simulink model "provaAttitude"  (R2023b)
settings: Solver=ode4  StartTime=t0  StopTime=tf  FixedStep=t_step  RelTol=1e-3
values from neighbouring files (symbols this model uses):
  A = 1e-2.*[6, 6, 6, 6, 4, 4, 12, 12, 12, 12]'    [provaAttitudeCode.m]
  A1 = ones(length(BODY),1)    [provaAttitudeCode.m]
  alpha = alpha/norm(alpha)    [provaAttitudeCode.m]
  BODY = [1, 0, 0 ... (first row only)    [provaAttitudeCode.m]
  c = 3e8    (= 300000000)    [provaAttitudeCode.m]
  DCM_eci_per = rotationMatrix(rad2deg(i),rad2deg(OM), rad2deg(om))    [provaAttitudeCode.m]
  e = 0.0001    [provaAttitudeCode.m]
  epsilon = deg2rad(23.45)    [provaAttitudeCode.m]
  Fe = 1358    [provaAttitudeCode.m]
  FS = 800e-9    (= 8e-07)    [provaAttitudeCode.m]
  H0 = 1e-9.*[-29404.8 -1450.9 4652.5]'    [provaAttitudeCode.m]
  horizon_cone_limit = deg2rad(67)    [provaAttitudeCode.m]
  i = deg2rad(90)    [provaAttitudeCode.m]
  I = [Ix, 0, 0; 0, Iy, 0; 0, 0, Iz]    [provaAttitudeCode.m]
  I_inv = inv(I)    [provaAttitudeCode.m]
  inc_tot = sqrt(inc_lin^2 + inc_acc^2)    [provaAttitudeCode.m]
  j_b = [0.01 0.05 0.01]'    [provaAttitudeCode.m]
  MJD2000_initial = date2mjd2000(date0)    [provaAttitudeCode.m]
  mu_E = astroConstants(13)    [provaAttitudeCode.m]
  n_e = sqrt(mu_E/a^3)    [provaAttitudeCode.m]
  p = a*(1-e^2)    [provaAttitudeCode.m]
  pd = 0.1.*A1    [provaAttitudeCode.m]
  ps = [0.5, 0.5, 0.5, 0.5, 0.5, 0.5, 0.1, 0.1, 0.1, 0.1]'    [provaAttitudeCode.m]
  q0 = [0 0 0 1]    [provaAttitudeCode.m]
  r1 = r(:,1) + CMC_position(1).*ones(10,1)    [provaAttitudeCode.m]
  r2 = r(:,2) + CMC_position(2).*ones(10,1)    [provaAttitudeCode.m]
  r3 = r(:,3)+ CMC_position(3).*ones(10,1)    [provaAttitudeCode.m]
  R_E = astroConstants(23)    [provaAttitudeCode.m]
  th0 = deg2rad(0)    [provaAttitudeCode.m]
  ts_sensor = t_step    (= 0.01)    [provaAttitudeCode.m]
  w0 = [wx0 wy0 wz0]'    [provaAttitudeCode.m]
  w_E = deg2rad(15.04)/60/60    [provaAttitudeCode.m]
  w_r = 0    [provaAttitudeCode.m]
libraries: matrix_library x16, dspindex x6, simulink_extras x4, simulink x3, aerolibutil x2
(part 1 of 2)
settings Model: Creator=samue  LastModifiedBy=samue

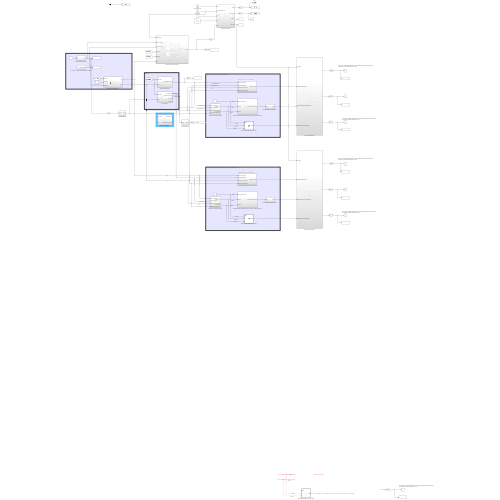
[thumbnail: Simulink's stored preview of the top-level diagram]
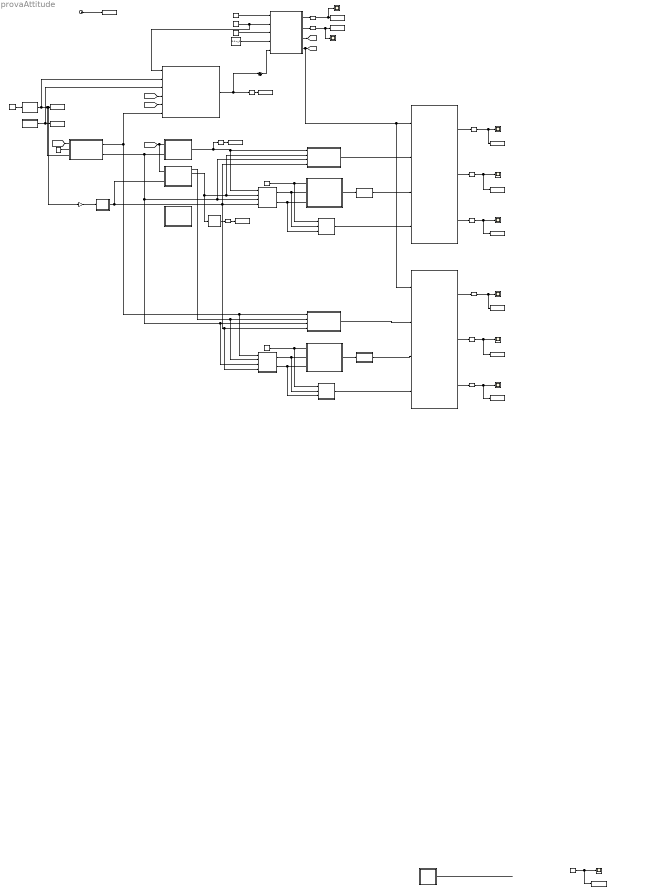
== system provaAttitude ==
  note: COMPARISON ATTITUDE DETERMINATION
  note: SENSOR
  note: Error from the real DCM and DCM att Det. If we eliminate the disturbance, sample holder and saturation we obtain estimate error of 1e-15
  note: Enviroment
  note: Error from the real DCM and DCM att Det. If we eliminate the disturbance, sample holder and saturation we obtain estimate error of 1e-11
  note: inside the block there is a normalisation
  note: UnPERTURBED CASE COMPARISON ATTITUDE DETERMINATION
  note: Error from the real DCM and DCM att Det. If we eliminate the disturbance, sample holder and saturation we obtain estimate error of 1e-11
  note: Error from the real DCM and DCM att Det. If we eliminate the disturbance, sample holder and saturation we obtain estimate error of 1e-15
  note: inside the block there is a normalisation
  note: Error from the real DCM and DCM att Det. If we eliminate the disturbance, sample holder and saturation we obtain estimate error of 1e-11
  Attitude determination algebric Method with 2 sensor : Subsystem
  Attitude determination algebric Method with 2 sensor1 : Subsystem
  Calculation of disturbance torque : Subsystem
  Clock : Clock
  Comparison (sottrazione) : Subsystem
  Comparison (sottrazione)1 : Subsystem
  Constant : Constant  Value=I_inv
  Constant1 : Constant  Value=alpha
  Constant2 : Constant  Value=[0,0,w_r]
  Constant3 : Constant  Value=alpha
  Constant4 : Constant  Value=th0
  Create matrix to statistical method : Subsystem
  Create matrix to statistical method1 : Subsystem
  DCM composition from quaternions 1 : Subsystem  AncestorBlock=LibrarySAD5/DCM composition from quaternions
  DCM composition from quaternions 2 : Subsystem  AncestorBlock=LibrarySAD5/DCM composition from quaternions
  Dipol Model of Magnetic Field : Subsystem
  Dynamics e Kinematics : Subsystem
  Gain : Gain  Gain=-1
  Horizon Sensor : Subsystem
  Inertia Matrix : Constant  Value=I  VectorParams1D=off
  Initial Condition W : Constant  Value=w0
  MAG-3  Magnetometer : Subsystem
  Normalize Vector1 : Subsystem
  Normalize Vector3 : Subsystem
  Ouput DCM with gibbs vector (ver slide) : MATLAB Function  TreatAsAtomicUnit=on
  Ouput DCM with gibbs vector (ver slide)1 : MATLAB Function  TreatAsAtomicUnit=on
  Ouput DCM with gibbs vector (ver slide)3 : MATLAB Function  TreatAsAtomicUnit=on
  Reshape{,1..10,17} (12 alike) : Reshape
  Scope{,1..7,10} (9 alike) : Scope
  "Statistical methods attitude determination (quaternion  Wabha’s problem) " : Subsystem
  Statistical methods attitude determination (quaternion  Wabha’s problem) 1 : Subsystem
  Sum : Sum  Inputs=|++
  Sun Position in Earth Centred Equatorial Inertial RF : Subsystem
  Sun sensor (Da fare) : Subsystem
  To Workspace : ToWorkspace  VariableName=r_n  SampleTime=-1
  To Workspace1 : ToWorkspace  VariableName=s_n  SampleTime=-1
  To Workspace10 : ToWorkspace  VariableName=erro_statistic_quat_unp  SampleTime=-1
  To Workspace11 : ToWorkspace  VariableName=erro_statistic_gibb_unp  SampleTime=-1
  To Workspace12 : ToWorkspace  VariableName=b_sensor  SampleTime=-1
  To Workspace13 : ToWorkspace  VariableName=sun_sensor  SampleTime=-1
  To Workspace15 : ToWorkspace  VariableName=erro_statistic_gibb_unp1  SampleTime=-1
  To Workspace2 : ToWorkspace  VariableName=wb  SampleTime=-1
  To Workspace3 : ToWorkspace  VariableName=M_dist  SaveFormat=Timeseries  SampleTime=-1
  To Workspace4 : ToWorkspace  VariableName=w  SampleTime=-1
  To Workspace5 : ToWorkspace  VariableName=erro_algebric_met  SampleTime=-1
  To Workspace6 : ToWorkspace  VariableName=erro_statistic_quat  SampleTime=-1
  To Workspace7 : ToWorkspace  VariableName=t  SampleTime=-1
  To Workspace8 : ToWorkspace  VariableName=erro_statistic_gibb  SampleTime=-1
  To Workspace9 : ToWorkspace  VariableName=erro_algebric_met_unp  SampleTime=-1
  "[g0_1, g1_1, h1_1]" : Constant  Value=H0
  two-body Keplerian dynamics : Subsystem
  wires:
  Constant2/1 -> Dynamics e Kinematics/4(w_r)
  Constant1/1 -> "Statistical methods attitude determination (quaternion  Wabha’s problem) "/1(alpha (weigh of sensor)), Ouput DCM with gibbs vector (ver slide)/1(alpha)  "alpha"
  two-body Keplerian dynamics/1(r_n) -> Calculation of disturbance torque/2(EarthSat_n vector), To Workspace/1, Gain/1, Dipol Model of Magnetic Field/3(EarthSat_n)
  [DCM_BN] -> Dipol Model of Magnetic Field/1(DCM_B/N)
  Sun Position in Earth Centred Equatorial Inertial RF/1(S_EarthSun_N) -> To Workspace1/1, Calculation of disturbance torque/3(SunEarth_n vector)  "S_n"
  Dipol Model of Magnetic Field/2(b_N) -> MAG-3  Magnetometer/2(B_N), Create matrix to statistical method/3(Reference1 (Inertial frame)), Attitude determination algebric Method with 2 sensor/3(Reference1 (Inertial frame)), Create matrix to statistical method1/3(Reference1 (Inertial frame)), Attitude determination algebric Method with 2 sensor1/3(Reference1 (Inertial frame))  "B_n"
  Reshape1/1 -> Scope7/1, To Workspace4/1
  Dipol Model of Magnetic Field/1(b_b) -> Create matrix to statistical method1/1(Sensor1 (body frame)), Attitude determination algebric Method with 2 sensor1/1(Sensor1 (body frame)), Calculation of disturbance torque/6(B_b)  "B_b"
  "[g0_1, g1_1, h1_1]"/1 -> Dipol Model of Magnetic Field/2(H0 vector)
  "Statistical methods attitude determination (quaternion  Wabha’s problem) "/1(q in quaternion (scalar last)) -> DCM composition from quaternions 1/1(q(4x1))
  [DCM_BN] -> Calculation of disturbance torque/5(DCM_B/N)
  [DCM_BL] -> Calculation of disturbance torque/4(DCM_B/L)
  MAG-3  Magnetometer/1(B_b perturbed sensor) -> Reshape9/1, Create matrix to statistical method/1(Sensor1 (body frame)), Attitude determination algebric Method with 2 sensor/1(Sensor1 (body frame))  "B_b perturbed sensor"
  [DCM_BN] -> Horizon Sensor/1(DCM_B/N), MAG-3  Magnetometer/1(DCM_B/N)
  Constant/1 -> Dynamics e Kinematics/3(I_inv)
  Calculation of disturbance torque/1(M_dist) -> Sum/1, Reshape2/1
  Constant4/1 -> two-body Keplerian dynamics/1(th0)
  Dynamics e Kinematics/1(Omega) -> Reshape1/1
  Clock/1 -> To Workspace7/1
  Reshape2/1 -> To Workspace3/1
  Initial Condition W/1 -> Dynamics e Kinematics/1(w0)
  Dynamics e Kinematics/3(DCM_B/L) -> [DCM_BL]
  Dynamics e Kinematics/2(Ang Vel Error) -> Reshape/1
  Inertia Matrix/1 -> Calculation of disturbance torque/1(Inertia Matrix), Dynamics e Kinematics/2("Principal Inertia Vector ")
  Reshape/1 -> Scope/1, To Workspace2/1
  Create matrix to statistical method/1(S matrix (body)) -> "Statistical methods attitude determination (quaternion  Wabha’s problem) "/2(s matrix), Ouput DCM with gibbs vector (ver slide)/2(s)  "S matrix"
  Create matrix to statistical method/2(V matrix (inertia)) -> "Statistical methods attitude determination (quaternion  Wabha’s problem) "/3(v matrix), Ouput DCM with gibbs vector (ver slide)/3(v)  "V matrix"
  Attitude determination algebric Method with 2 sensor/1(DCM_B/N  Att Det) -> Comparison (sottrazione)/2(DCM from Algebric method)
  DCM composition from quaternions 1/1(DCM) -> Comparison (sottrazione)/3("DCM from Statistic method (quaternion) ")
  Ouput DCM with gibbs vector (ver slide)/1(DCM) -> Comparison (sottrazione)/4("DCM from Statistic method (gibbs) ")
  Comparison (sottrazione)/1(Out1) -> Reshape3/1
  Comparison (sottrazione)/2(Out2) -> Reshape4/1
  Comparison (sottrazione)/3(Out3) -> Reshape5/1
  Reshape3/1 -> To Workspace5/1, Scope3/1
  Reshape4/1 -> To Workspace6/1, Scope2/1
  Reshape5/1 -> To Workspace8/1, Scope1/1
  Create matrix to statistical method1/1(S matrix (body)) -> Statistical methods attitude determination (quaternion  Wabha’s problem) 1/2(s matrix), Ouput DCM with gibbs vector (ver slide)1/2(s)  "S matrix"
  Create matrix to statistical method1/2(V matrix (inertia)) -> Statistical methods attitude determination (quaternion  Wabha’s problem) 1/3(v matrix), Ouput DCM with gibbs vector (ver slide)1/3(v)  "V matrix"
  Comparison (sottrazione)1/3(Out3) -> Reshape8/1
  Dynamics e Kinematics/4(DCM_B/N) -> Comparison (sottrazione)1/1(True DCM), Comparison (sottrazione)/1(True DCM), [DCM_BN]
  Attitude determination algebric Method with 2 sensor1/1(DCM_B/N  Att Det) -> Comparison (sottrazione)1/2(DCM from Algebric method)
  Comparison (sottrazione)1/2(Out2) -> Reshape7/1
  Ouput DCM with gibbs vector (ver slide)1/1(DCM) -> Comparison (sottrazione)1/4("DCM from Statistic method (gibbs) ")
  DCM composition from quaternions 2/1(DCM) -> Comparison (sottrazione)1/3("DCM from Statistic method (quaternion) ")
  Comparison (sottrazione)1/1(Out1) -> Reshape6/1
  Reshape7/1 -> To Workspace10/1, Scope5/1
  Constant3/1 -> Statistical methods attitude determination (quaternion  Wabha’s problem) 1/1(alpha (weigh of sensor)), Ouput DCM with gibbs vector (ver slide)1/1(alpha)  "alpha"
  Reshape6/1 -> To Workspace9/1, Scope6/1
  Statistical methods attitude determination (quaternion  Wabha’s problem) 1/1(q in quaternion (scalar last)) -> DCM composition from quaternions 2/1(q(4x1))
  Reshape8/1 -> To Workspace11/1, Scope4/1
  Reshape9/1 -> To Workspace12/1
  Horizon Sensor/2(Perturbed data Horizon) -> Normalize Vector1/1(Vector), Attitude determination algebric Method with 2 sensor/2(Sensor2 (body frame)), Create matrix to statistical method/2(Sensor2 (body frame))  "S_b perturbed sensor"
  Horizon Sensor/1(R_b unperturbed) -> Create matrix to statistical method1/2(Sensor2 (body frame)), Attitude determination algebric Method with 2 sensor1/2(Sensor2 (body frame))  "S_b unperturbed"
  Reshape10/1 -> To Workspace13/1
  Normalize Vector1/1(Versor) -> Reshape10/1
  Reshape17/1 -> To Workspace15/1, Scope10/1
  ? -> Ouput DCM with gibbs vector (ver slide)3/2(s)  "S matrix"
  ? -> ?
  ? -> Reshape17/1
  Ouput DCM with gibbs vector (ver slide)3/1(DCM) -> ?
  ? -> Ouput DCM with gibbs vector (ver slide)3/3(v)  "V matrix"
  Gain/1 -> Normalize Vector3/1(Vector)
  Normalize Vector3/1(Versor) -> Horizon Sensor/2(R_N), Create matrix to statistical method/4(Reference2 (Inertial frame)), Attitude determination algebric Method with 2 sensor/4(Reference2 (Inertial frame)), Create matrix to statistical method1/4(Reference2 (Inertial frame)), Attitude determination algebric Method with 2 sensor1/4(Reference2 (Inertial frame))
  Sum/1 -> Dynamics e Kinematics/5(M)

== system provaAttitude/Attitude determination algebric Method with 2 sensor ==
  note: 𝑉^(-1) = 𝑉';
      | 𝐴 = 𝑆𝑉^(-1) = 𝑆𝑉'
  note: 𝑣1 = 𝑎;
      | 𝑣2 = (𝑎 ∧ 𝑏)/|𝑎 ∧ 𝑏|;
      | 𝑣3 = 𝑎 ∧ 𝑣2
  note: S1 = 𝑝;
      | 𝑠2 = (𝑝 ∧ 𝑞)/(|𝑝 ∧ 𝑞|);
      | 𝑠3 = 𝑝 ∧ 𝑠2
  Sensor1 (body frame) : Inport
  Sensor2 (body frame) : Inport  Port=2
  Reference1 (Inertial frame) : Inport  Port=3
  Reference2 (Inertial frame) : Inport  Port=4
  Matrix Multiply : Product  Multiplication=Matrix(*)
  Normalize Vector1 : Subsystem
  Normalize Vector2 : Subsystem
  Normalize Vector3 : Subsystem
  Normalize Vector4 : Subsystem
  Subsystem : Subsystem
  Subsystem1 : Subsystem
  Transpose : Math  Operator=transpose
  DCM_B/N  Att Det : Outport
  wires:
  Sensor1 (body frame)/1 -> Normalize Vector2/1(Vector)  "q"
  Sensor2 (body frame)/1 -> Normalize Vector3/1(Vector)  "p"
  Subsystem/1("Matrix S Measurements ") -> Matrix Multiply/1  "Matrix S Measurements (body frame)"
  Normalize Vector2/1(Versor) -> Subsystem/1(versor p (body frame))
  Normalize Vector3/1(Versor) -> Subsystem/2(versor q (body frame))
  Normalize Vector1/1(Versor) -> Subsystem1/1(versor a (body frame))
  Reference2 (Inertial frame)/1 -> Normalize Vector4/1(Vector)  "b"
  Reference1 (Inertial frame)/1 -> Normalize Vector1/1(Vector)  "a"
  Subsystem1/1("Matrix V certain model ") -> Transpose/1  "Matrix V (inertial frame)"
  Normalize Vector4/1(Versor) -> Subsystem1/2(versor b (body frame))
  Matrix Multiply/1 -> DCM_B/N  Att Det/1  "DCM_B/N from attirude determination"
  Transpose/1 -> Matrix Multiply/2

== system provaAttitude/Attitude determination algebric Method with 2 sensor1 ==
  note: 𝑉^(-1) = 𝑉';
      | 𝐴 = 𝑆𝑉^(-1) = 𝑆𝑉'
  note: 𝑣1 = 𝑎;
      | 𝑣2 = (𝑎 ∧ 𝑏)/|𝑎 ∧ 𝑏|;
      | 𝑣3 = 𝑎 ∧ 𝑣2
  note: S1 = 𝑝;
      | 𝑠2 = (𝑝 ∧ 𝑞)/(|𝑝 ∧ 𝑞|);
      | 𝑠3 = 𝑝 ∧ 𝑠2
  Sensor1 (body frame) : Inport
  Sensor2 (body frame) : Inport  Port=2
  Reference1 (Inertial frame) : Inport  Port=3
  Reference2 (Inertial frame) : Inport  Port=4
  Matrix Multiply : Product  Multiplication=Matrix(*)
  Normalize Vector1 : Subsystem
  Normalize Vector2 : Subsystem
  Normalize Vector3 : Subsystem
  Normalize Vector4 : Subsystem
  Subsystem : Subsystem
  Subsystem1 : Subsystem
  Transpose : Math  Operator=transpose
  DCM_B/N  Att Det : Outport
  wires:
  Sensor1 (body frame)/1 -> Normalize Vector2/1(Vector)  "q"
  Sensor2 (body frame)/1 -> Normalize Vector3/1(Vector)  "p"
  Subsystem/1("Matrix S Measurements ") -> Matrix Multiply/1  "Matrix S Measurements (body frame)"
  Normalize Vector2/1(Versor) -> Subsystem/1(versor p (body frame))
  Normalize Vector3/1(Versor) -> Subsystem/2(versor q (body frame))
  Normalize Vector1/1(Versor) -> Subsystem1/1(versor a (body frame))
  Reference2 (Inertial frame)/1 -> Normalize Vector4/1(Vector)  "b"
  Reference1 (Inertial frame)/1 -> Normalize Vector1/1(Vector)  "a"
  Subsystem1/1("Matrix V certain model ") -> Transpose/1  "Matrix V (inertial frame)"
  Normalize Vector4/1(Versor) -> Subsystem1/2(versor b (body frame))
  Matrix Multiply/1 -> DCM_B/N  Att Det/1  "DCM_B/N from attirude determination"
  Transpose/1 -> Matrix Multiply/2

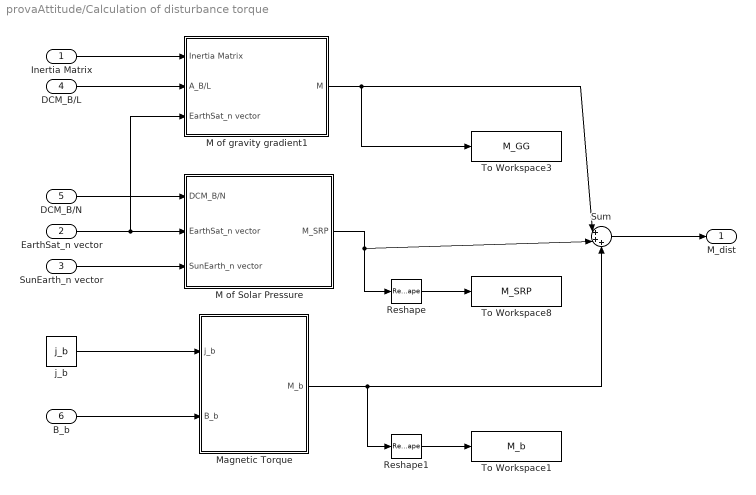
== system provaAttitude/Calculation of disturbance torque ==
  Inertia Matrix : Inport
  EarthSat_n vector : Inport  Port=2
  SunEarth_n vector : Inport  Port=3
  DCM_B/L : Inport  Port=4
  DCM_B/N : Inport  Port=5
  B_b : Inport  Port=6
  M of Solar Pressure : Subsystem
  M of gravity gradient1 : Subsystem
  Magnetic Torque : Subsystem
  Reshape : Reshape
  Reshape1 : Reshape
  Sum : Sum  Inputs=|+++
  To Workspace1 : ToWorkspace  VariableName=M_b  SampleTime=-1
  To Workspace3 : ToWorkspace  VariableName=M_GG  SampleTime=-1
  To Workspace8 : ToWorkspace  VariableName=M_SRP  SampleTime=-1
  j_b : Constant  Value=j_b
  M_dist : Outport
  wires:
  DCM_B/L/1 -> M of gravity gradient1/2(A_B/L)
  j_b/1 -> Magnetic Torque/1(j_b)
  Magnetic Torque/1(M_b) -> Sum/3, Reshape1/1
  B_b/1 -> Magnetic Torque/2(B_b)
  Inertia Matrix/1 -> M of gravity gradient1/1(Inertia Matrix)
  M of Solar Pressure/1(M_SRP) -> Sum/2, Reshape/1
  EarthSat_n vector/1 -> M of gravity gradient1/3(EarthSat_n vector), M of Solar Pressure/2(EarthSat_n vector)
  DCM_B/N/1 -> M of Solar Pressure/1(DCM_B/N)
  SunEarth_n vector/1 -> M of Solar Pressure/3(SunEarth_n vector)
  Sum/1 -> M_dist/1
  Reshape/1 -> To Workspace8/1
  Reshape1/1 -> To Workspace1/1
  M of gravity gradient1/1(M) -> To Workspace3/1, Sum/1

== system provaAttitude/Comparison (sottrazione) ==
  True DCM : Inport
  DCM from Algebric method : Inport  Port=2
  "DCM from Statistic method (quaternion) " : Inport  Port=3
  "DCM from Statistic method (gibbs) " : Inport  Port=4
  Matrix Sum : Sum  Inputs=+
  Matrix Sum1 : Sum  Inputs=+
  Matrix Sum2 : Sum  Inputs=+
  Sum : Sum  Inputs=|+-
  Sum1 : Sum  Inputs=|+-
  Sum2 : Sum  Inputs=|+-
  Out1 : Outport
  Out2 : Outport  Port=2
  Out3 : Outport  Port=3
  wires:
  "DCM from Statistic method (quaternion) "/1 -> Sum1/1
  True DCM/1 -> Sum/2, Sum1/2, Sum2/2
  Sum1/1 -> Matrix Sum1/1
  Sum/1 -> Matrix Sum/1
  "DCM from Statistic method (gibbs) "/1 -> Sum/1
  Sum2/1 -> Matrix Sum2/1
  Matrix Sum1/1 -> Out2/1
  Matrix Sum/1 -> Out3/1
  DCM from Algebric method/1 -> Sum2/1
  Matrix Sum2/1 -> Out1/1

== system provaAttitude/Comparison (sottrazione)1 ==
  True DCM : Inport
  DCM from Algebric method : Inport  Port=2
  "DCM from Statistic method (quaternion) " : Inport  Port=3
  "DCM from Statistic method (gibbs) " : Inport  Port=4
  Matrix Sum : Sum  Inputs=+
  Matrix Sum1 : Sum  Inputs=+
  Matrix Sum2 : Sum  Inputs=+
  Sum : Sum  Inputs=|+-
  Sum1 : Sum  Inputs=|+-
  Sum2 : Sum  Inputs=|+-
  Out1 : Outport
  Out2 : Outport  Port=2
  Out3 : Outport  Port=3
  wires:
  "DCM from Statistic method (quaternion) "/1 -> Sum1/1
  True DCM/1 -> Sum/2, Sum1/2, Sum2/2
  Sum1/1 -> Matrix Sum1/1
  Sum/1 -> Matrix Sum/1
  "DCM from Statistic method (gibbs) "/1 -> Sum/1
  Sum2/1 -> Matrix Sum2/1
  Matrix Sum1/1 -> Out2/1
  Matrix Sum/1 -> Out3/1
  DCM from Algebric method/1 -> Sum2/1
  Matrix Sum2/1 -> Out1/1

== system provaAttitude/Create matrix to statistical method ==
  Sensor1 (body frame) : Inport
  Sensor2 (body frame) : Inport  Port=2
  Reference1 (Inertial frame) : Inport  Port=3
  Reference2 (Inertial frame) : Inport  Port=4
  Matrix Concatenate1 : Concatenate  Mode=Multidimensional array  ConcatenateDimension=2
  Matrix Concatenate2 : Concatenate  Mode=Multidimensional array  ConcatenateDimension=2
  Normalize Vector1 : Subsystem
  Normalize Vector2 : Subsystem
  Normalize Vector3 : Subsystem
  Normalize Vector4 : Subsystem
  S matrix (body) : Outport
  V matrix (inertia) : Outport  Port=2
  wires:
  Matrix Concatenate1/1 -> V matrix (inertia)/1
  Normalize Vector1/1(Versor) -> Matrix Concatenate2/1
  Normalize Vector2/1(Versor) -> Matrix Concatenate2/2
  Normalize Vector4/1(Versor) -> Matrix Concatenate1/2
  Normalize Vector3/1(Versor) -> Matrix Concatenate1/1
  Matrix Concatenate2/1 -> S matrix (body)/1
  Reference1 (Inertial frame)/1 -> Normalize Vector3/1(Vector)
  Reference2 (Inertial frame)/1 -> Normalize Vector4/1(Vector)
  Sensor1 (body frame)/1 -> Normalize Vector1/1(Vector)
  Sensor2 (body frame)/1 -> Normalize Vector2/1(Vector)

== system provaAttitude/Create matrix to statistical method1 ==
  Sensor1 (body frame) : Inport
  Sensor2 (body frame) : Inport  Port=2
  Reference1 (Inertial frame) : Inport  Port=3
  Reference2 (Inertial frame) : Inport  Port=4
  Matrix Concatenate1 : Concatenate  Mode=Multidimensional array  ConcatenateDimension=2
  Matrix Concatenate2 : Concatenate  Mode=Multidimensional array  ConcatenateDimension=2
  Normalize Vector1 : Subsystem
  Normalize Vector2 : Subsystem
  Normalize Vector3 : Subsystem
  Normalize Vector4 : Subsystem
  S matrix (body) : Outport
  V matrix (inertia) : Outport  Port=2
  wires:
  Matrix Concatenate1/1 -> V matrix (inertia)/1
  Normalize Vector1/1(Versor) -> Matrix Concatenate2/1
  Normalize Vector2/1(Versor) -> Matrix Concatenate2/2
  Normalize Vector4/1(Versor) -> Matrix Concatenate1/2
  Normalize Vector3/1(Versor) -> Matrix Concatenate1/1
  Matrix Concatenate2/1 -> S matrix (body)/1
  Reference1 (Inertial frame)/1 -> Normalize Vector3/1(Vector)
  Reference2 (Inertial frame)/1 -> Normalize Vector4/1(Vector)
  Sensor1 (body frame)/1 -> Normalize Vector1/1(Vector)
  Sensor2 (body frame)/1 -> Normalize Vector2/1(Vector)

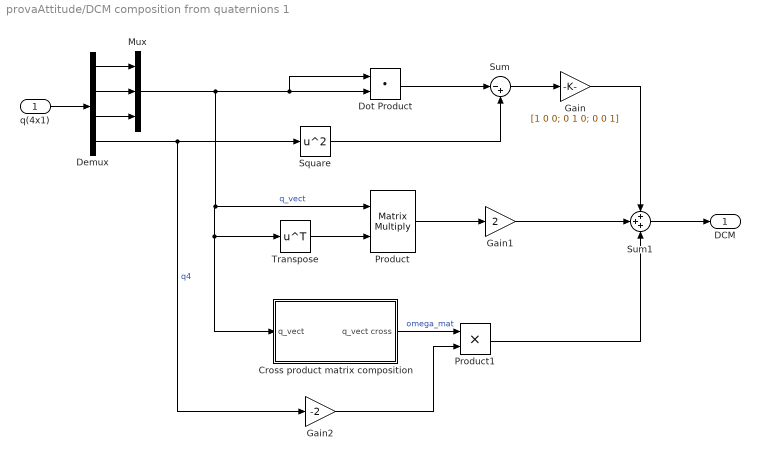
== system provaAttitude/DCM composition from quaternions 1 ==
  q(4x1) : Inport
  Cross product matrix composition : Subsystem
  Demux : Demux
  Dot Product : DotProduct  OutDataTypeStr=Inherit: Inherit via internal rule
  Gain : Gain  Gain=[1 0 0; 0 1 0; 0 0 1]
  Gain1 : Gain  Gain=2
  Gain2 : Gain  Gain=-2
  Mux : Mux  Inputs=3
  Product : Product  Multiplication=Matrix(*)
  Product1 : Product
  Square : Math  Operator=square
  Sum : Sum  Inputs=|-+
  Sum1 : Sum  Inputs=+++
  Transpose : Math  Operator=transpose
  DCM : Outport
  wires:
  Gain/1 -> Sum1/1
  Demux/1 -> Mux/1
  q(4x1)/1 -> Demux/1
  Demux/2 -> Mux/2
  Mux/1 -> Dot Product/2, Dot Product/1, Product/1, Cross product matrix composition/1(q_vect), Transpose/1  "q_vect"
  Demux/4 -> Gain2/1, Square/1  "q4"
  Demux/3 -> Mux/3
  Dot Product/1 -> Sum/1
  Sum/1 -> Gain/1
  Square/1 -> Sum/2
  Transpose/1 -> Product/2
  Product/1 -> Gain1/1
  Gain2/1 -> Product1/2
  Cross product matrix composition/1(q_vect cross) -> Product1/1  "omega_mat"
  Product1/1 -> Sum1/3
  Gain1/1 -> Sum1/2
  Sum1/1 -> DCM/1

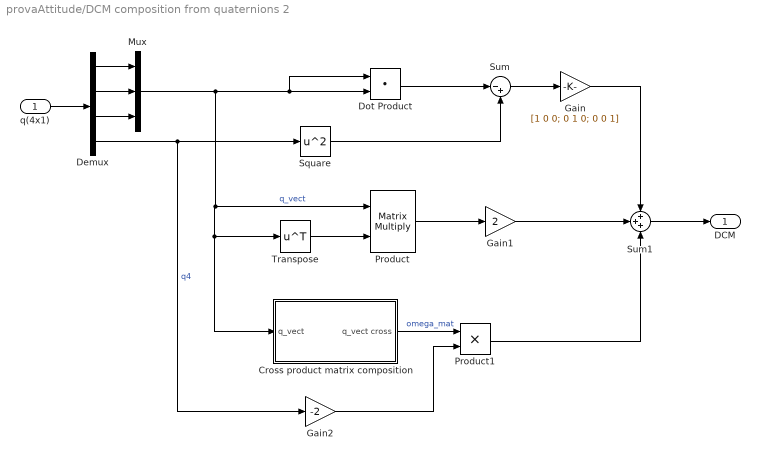
== system provaAttitude/DCM composition from quaternions 2 ==
  q(4x1) : Inport
  Cross product matrix composition : Subsystem
  Demux : Demux
  Dot Product : DotProduct  OutDataTypeStr=Inherit: Inherit via internal rule
  Gain : Gain  Gain=[1 0 0; 0 1 0; 0 0 1]
  Gain1 : Gain  Gain=2
  Gain2 : Gain  Gain=-2
  Mux : Mux  Inputs=3
  Product : Product  Multiplication=Matrix(*)
  Product1 : Product
  Square : Math  Operator=square
  Sum : Sum  Inputs=|-+
  Sum1 : Sum  Inputs=+++
  Transpose : Math  Operator=transpose
  DCM : Outport
  wires:
  Gain/1 -> Sum1/1
  Demux/1 -> Mux/1
  q(4x1)/1 -> Demux/1
  Demux/2 -> Mux/2
  Mux/1 -> Dot Product/2, Dot Product/1, Product/1, Cross product matrix composition/1(q_vect), Transpose/1  "q_vect"
  Demux/4 -> Gain2/1, Square/1  "q4"
  Demux/3 -> Mux/3
  Dot Product/1 -> Sum/1
  Sum/1 -> Gain/1
  Square/1 -> Sum/2
  Transpose/1 -> Product/2
  Product/1 -> Gain1/1
  Gain2/1 -> Product1/2
  Cross product matrix composition/1(q_vect cross) -> Product1/1  "omega_mat"
  Product1/1 -> Sum1/3
  Gain1/1 -> Sum1/2
  Sum1/1 -> DCM/1

== system provaAttitude/Dipol Model of Magnetic Field ==
  note: CODE TO ADD
      | % Definition of Magnetic Field (Dipole model)
      |  j_b = [0.01 0.05 0.01]';
      | H0 = 1e-9.*[-29404.8 -1450.9 4652.5]';
  DCM_B/N : Inport
  H0 vector : Inport  Port=2
  EarthSat_n : Inport  Port=3
  Calculation of b_n : Subsystem
  Matrix Multiply : Product  Multiplication=Matrix(*)
  To Workspace : ToWorkspace  VariableName=bn  SampleTime=-1
  b_b : Outport
  b_N : Outport  Port=2
  wires:
  Matrix Multiply/1 -> b_b/1
  DCM_B/N/1 -> Matrix Multiply/1
  H0 vector/1 -> Calculation of b_n/1(H0 vector)
  EarthSat_n/1 -> Calculation of b_n/2(EarthSat_n)
  Calculation of b_n/1(b_N) -> Matrix Multiply/2, To Workspace/1, b_N/1

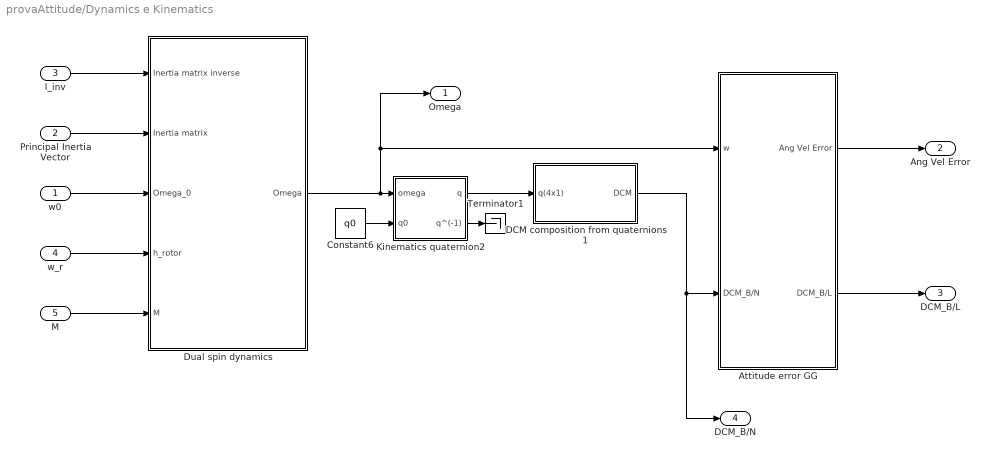
== system provaAttitude/Dynamics e Kinematics ==
  w0 : Inport
  "Principal Inertia Vector " : Inport  Port=2
  I_inv : Inport  Port=3
  w_r : Inport  Port=4
  M : Inport  Port=5
  Attitude error GG : Subsystem
  Constant6 : Constant  Value=q0
  DCM composition from quaternions 1 : Subsystem  AncestorBlock=LibrarySAD5/DCM composition from quaternions
  Dual spin dynamics : Subsystem  AncestorBlock=LibrarySAD5/Dual spin dynamics
  Kinematics quaternion2 : Subsystem
  Terminator1 : Terminator
  Omega : Outport
  Ang Vel Error : Outport  Port=2
  DCM_B/L : Outport  Port=3
  DCM_B/N : Outport  Port=4
  wires:
  DCM composition from quaternions 1/1(DCM) -> DCM_B/N/1, Attitude error GG/2(DCM_B/N)
  Constant6/1 -> Kinematics quaternion2/2(q0)
  Dual spin dynamics/1(Omega) -> Omega/1, Attitude error GG/1(w), Kinematics quaternion2/1(omega)
  Kinematics quaternion2/2(q^(-1)) -> Terminator1/1
  M/1 -> Dual spin dynamics/5(M)
  w0/1 -> Dual spin dynamics/3(Omega_0)
  "Principal Inertia Vector "/1 -> Dual spin dynamics/2(Inertia matrix)
  Kinematics quaternion2/1(q) -> DCM composition from quaternions 1/1(q(4x1))
  Attitude error GG/2(DCM_B/L) -> DCM_B/L/1
  Attitude error GG/1(Ang Vel Error) -> Ang Vel Error/1
  I_inv/1 -> Dual spin dynamics/1(Inertia matrix inverse)
  w_r/1 -> Dual spin dynamics/4(h_rotor)

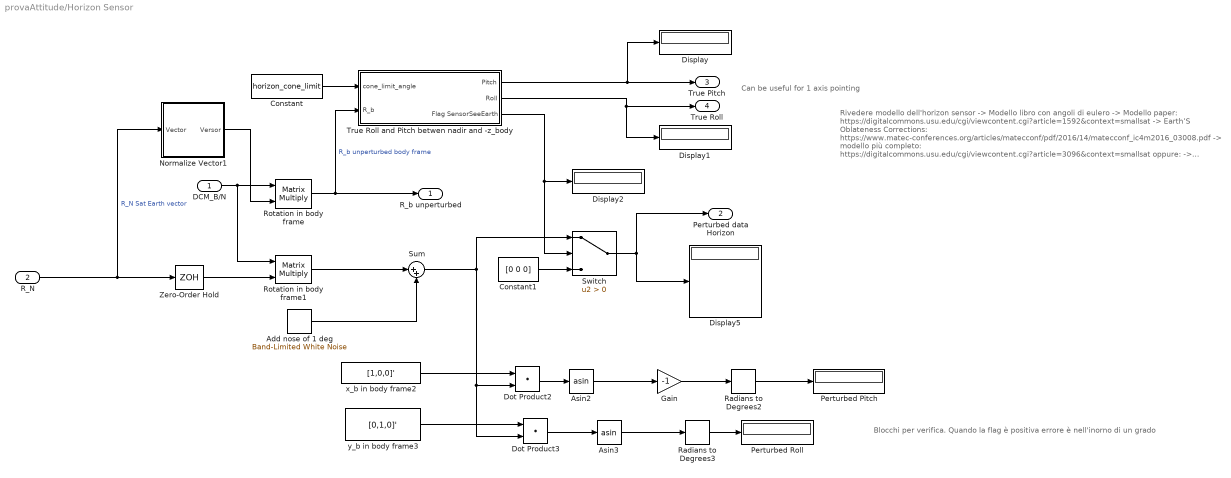
== system provaAttitude/Horizon Sensor ==
  note: Can be useful for 1 axis pointing
  note: Rivedere modello dell'horizon sensor
      | -> Modello libro con angoli di eulero
      | -> Modello paper: https://digitalcommons.usu.edu/cgi/viewcontent.cgi?article=1592&context=smallsat
      | -> Earth’S Oblateness Corrections: https://www.matec-conferences.org/articles/matecconf/pdf/2016/14/matecconf_ic4m2016_03008.pdf
      | -> modello più completo: https://digitalcommons.usu.edu/cgi/viewcontent.cgi?article=3096&context=smallsat
      | oppure:
      | -> Sistemare errore in modo che non sia lineare
      | -> Controllare angoli e conversioni
  note: Blocchi per verifica. Quando la flag è positiva errore è nell'inorno di un grado
  DCM_B/N : Inport
  R_N : Inport  Port=2
  Add nose of 1 deg : simulink/Sources/Band-Limited White Noise  Cov=[0.000001 0.000001 0]  Ts=ts_sensor  seed=[23341]
  Asin2 : Trigonometry  Operator=asin
  Asin3 : Trigonometry  Operator=asin
  Constant : Constant  Value=horizon_cone_limit
  Constant1 : Constant  Value=[0 0 0]
  Display{,1..2,5} (4 alike) : Display
  Dot Product2 : DotProduct  OutDataTypeStr=Inherit: Inherit via internal rule
  Dot Product3 : DotProduct  OutDataTypeStr=Inherit: Inherit via internal rule
  Gain : Gain  Gain=-1
  Normalize Vector1 : Subsystem
  Perturbed Pitch : Display
  Perturbed Roll : Display
  Radians to Degrees2 : simulink_extras/Transformations/Radians to Degrees
  Radians to Degrees3 : simulink_extras/Transformations/Radians to Degrees
  Rotation in body frame : Product  Multiplication=Matrix(*)
  Rotation in body frame1 : Product  Multiplication=Matrix(*)
  Sum : Sum  Inputs=|++
  Switch : Switch  Criteria=u2 > Threshold  SaturateOnIntegerOverflow=off  InputSameDT=off
  True Roll and Pitch betwen nadir and -z_body : Subsystem
  Zero-Order Hold : ZeroOrderHold  SampleTime=ts_sensor
  x_b in body frame2 : Constant  Value=[1,0,0]'
  y_b in body frame3 : Constant  Value=[0,1,0]'
  R_b unperturbed : Outport
  Perturbed data Horizon : Outport  Port=2
  True Pitch : Outport  Port=3
  True Roll : Outport  Port=4
  wires:
  y_b in body frame3/1 -> Dot Product3/1
  Zero-Order Hold/1 -> Rotation in body frame1/2
  True Roll and Pitch betwen nadir and -z_body/3(Flag SensorSeeEarth) -> Switch/2, Display2/1
  Normalize Vector1/1(Versor) -> Rotation in body frame/2
  R_N/1 -> Zero-Order Hold/1, Normalize Vector1/1(Vector)  "R_N Sat Earth vector"
  Rotation in body frame1/1 -> Sum/1
  Asin2/1 -> Gain/1
  DCM_B/N/1 -> Rotation in body frame/1, Rotation in body frame1/1
  Switch/1 -> Perturbed data Horizon/1, Display5/1
  True Roll and Pitch betwen nadir and -z_body/1(Pitch) -> Display/1, True Pitch/1
  Constant/1 -> True Roll and Pitch betwen nadir and -z_body/1(cone_limit_angle)
  Dot Product2/1 -> Asin2/1
  Rotation in body frame/1 -> R_b unperturbed/1, True Roll and Pitch betwen nadir and -z_body/2(R_b)  "R_b unperturbed body frame"
  Add nose of 1 deg/1 -> Sum/2
  True Roll and Pitch betwen nadir and -z_body/2(Roll) -> Display1/1, True Roll/1
  x_b in body frame2/1 -> Dot Product2/1
  Radians to Degrees2/1 -> Perturbed Pitch/1
  Sum/1 -> Switch/1, Dot Product2/2, Dot Product3/2
  Dot Product3/1 -> Asin3/1
  Asin3/1 -> Radians to Degrees3/1
  Gain/1 -> Radians to Degrees2/1
  Radians to Degrees3/1 -> Perturbed Roll/1
  Constant1/1 -> Switch/3

== system provaAttitude/MAG-3  Magnetometer ==
  note: CODE TO ADD TO MAKE SENSOR WORK
      | % Time definition
      | t0 = 0;
      | tf = T; %Period of orbit
      | t_step = 0.01; %fixed step of simulation
      | ts_sensor = t_step; % Sample of sensor (can change but must to be a multiple of t_step)
      |
      | % MAG-3 sensor data and error
      | FS = 500e-9; %Full scale value
      | inc_lin = 0.15/100; % Accuracy error
      | inc_acc = 0.75/100; % Linear error
      | inc_tot = sqrt(inc_lin^2 + inc_acc^2); %Total error
  DCM_B/N : Inport
  B_N : Inport  Port=2
  Error gain of sensor MAG-3 : Gain  Gain=inc_tot*FS
  Rotation in body frame : Product  Multiplication=Matrix(*)
  Saturation to FS : Saturate  UpperLimit=FS  LowerLimit=-FS
  Sum : Sum  Inputs=|++
  Vector Concatenate : Concatenate  NumInputs=3
  White Noise : RandomNumber  DisableCoverage=on  Seed=1  SampleTime=ts_sensor
  White Noise1 : RandomNumber  DisableCoverage=on  Seed=2  SampleTime=ts_sensor
  White Noise2 : RandomNumber  DisableCoverage=on  Seed=3  SampleTime=ts_sensor
  Zero-Order Hold : ZeroOrderHold  SampleTime=ts_sensor
  B_b perturbed sensor : Outport
  wires:
  Vector Concatenate/1 -> Error gain of sensor MAG-3/1
  White Noise/1 -> Vector Concatenate/1
  Error gain of sensor MAG-3/1 -> Sum/2
  White Noise2/1 -> Vector Concatenate/3
  White Noise1/1 -> Vector Concatenate/2
  DCM_B/N/1 -> Rotation in body frame/1
  B_N/1 -> Zero-Order Hold/1
  Zero-Order Hold/1 -> Rotation in body frame/2
  Saturation to FS/1 -> B_b perturbed sensor/1
  Rotation in body frame/1 -> Sum/1
  Sum/1 -> Saturation to FS/1

== system provaAttitude/Normalize Vector1 ==
  Vector : Inport
  Divide : Product  Inputs=*/
  Normalize Vector : Subsystem  AncestorBlock=LibrarySAD5/Normalize Vector1
  Versor : Outport
  wires:
  Vector/1 -> Normalize Vector/1(Vector), Divide/1
  Divide/1 -> Versor/1
  Normalize Vector/1(Norm) -> Divide/2

== system provaAttitude/Normalize Vector3 ==
  Vector : Inport
  Divide : Product  Inputs=*/
  Normalize Vector : Subsystem  AncestorBlock=LibrarySAD5/Normalize Vector1
  Versor : Outport
  wires:
  Vector/1 -> Normalize Vector/1(Vector), Divide/1
  Divide/1 -> Versor/1
  Normalize Vector/1(Norm) -> Divide/2

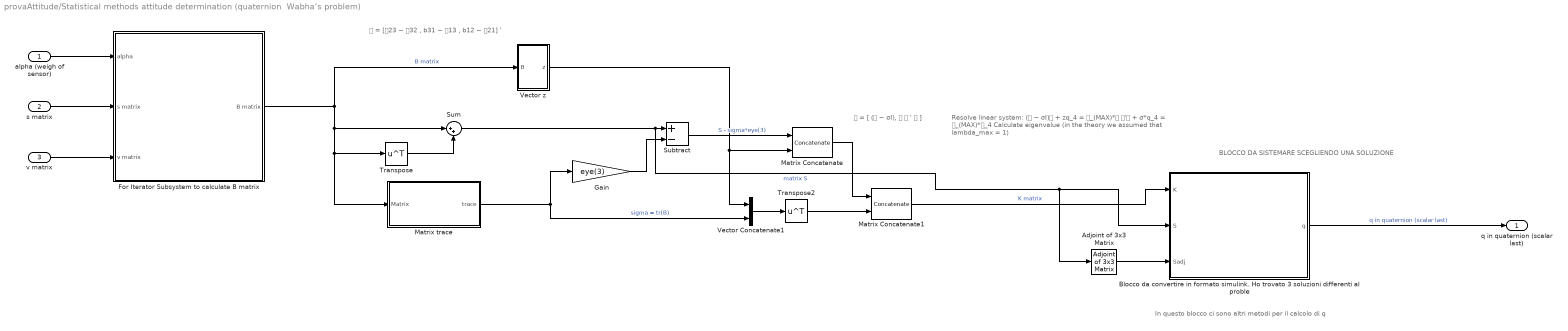
== system provaAttitude/Statistical methods attitude determination (quaternion  Wabha’s problem)  ==
  note: In questo blocco ci sono altri metodi per il calcolo di q
  note: BLOCCO DA SISTEMARE SCEGLIENDO UNA SOLUZIONE
  note: Resolve linear system:
      | (𝑆 − σI)𝑞 + zq_4 = 𝜆_(MAX)*𝑞
      | 𝑧'𝑞 + σ*q_4 = 𝜆_(MAX)*𝑞_4
      |
      | Calculate eigenvalue (in the theory we assumed that lambda_max = 1)
  note: 𝐾 = [ (𝑆 − σI), 𝑧
      | 𝑧 ' 𝜎 ]
  note: 𝑧 = [𝑏23 − 𝑏32 , b31 − 𝑏13 , b12 − 𝑏21] '
  alpha (weigh of sensor) : Inport
  s matrix : Inport  Port=2
  v matrix : Inport  Port=3
  Adjoint of 3x3 Matrix : aerolibutil/Adjoint of 3x3 Matrix
  Blocco da convertire in formato simulink. Ho trovato 3 soluzioni differenti al proble : MATLAB Function  TreatAsAtomicUnit=on
  For Iterator Subsystem to calculate B matrix : Subsystem  TreatAsAtomicUnit=on
  Gain : Gain  Gain=eye(3)
  Matrix Concatenate : Concatenate  Mode=Multidimensional array  ConcatenateDimension=2
  Matrix Concatenate1 : Concatenate  Mode=Multidimensional array
  Matrix trace : Subsystem
  Subtract : Sum  Inputs=+-
  Sum : Sum  Inputs=|++
  Transpose : Math  Operator=transpose
  Transpose2 : Math  Operator=transpose
  Vector Concatenate1 : Concatenate
  Vector z : Subsystem
  q in quaternion (scalar last) : Outport
  wires:
  Transpose/1 -> Sum/2
  For Iterator Subsystem to calculate B matrix/1(B matrix) -> Vector z/1(B), Matrix trace/1(Matrix), Transpose/1, Sum/1  "B matrix"
  Sum/1 -> Adjoint of 3x3 Matrix/1, Blocco da convertire in formato simulink. Ho trovato 3 soluzioni differenti al proble/2(S), Subtract/1  "matrix S"
  Gain/1 -> Subtract/2
  Matrix trace/1(trace) -> Vector Concatenate1/2, Gain/1  "sigma = tr(B)"
  Matrix Concatenate/1 -> Matrix Concatenate1/1
  Vector Concatenate1/1 -> Transpose2/1
  Vector z/1(z) -> Vector Concatenate1/1, Matrix Concatenate/2
  Transpose2/1 -> Matrix Concatenate1/2
  Subtract/1 -> Matrix Concatenate/1  "S - sigma*eye(3)"
  alpha (weigh of sensor)/1 -> For Iterator Subsystem to calculate B matrix/1(alpha)
  v matrix/1 -> For Iterator Subsystem to calculate B matrix/3(v matrix)
  s matrix/1 -> For Iterator Subsystem to calculate B matrix/2(s matrix)
  Blocco da convertire in formato simulink. Ho trovato 3 soluzioni differenti al proble/1(q) -> q in quaternion (scalar last)/1  "q in quaternion (scalar last)"
  Adjoint of 3x3 Matrix/1 -> Blocco da convertire in formato simulink. Ho trovato 3 soluzioni differenti al proble/3(Sadj)
  Matrix Concatenate1/1 -> Blocco da convertire in formato simulink. Ho trovato 3 soluzioni differenti al proble/1(K)  "K matrix"

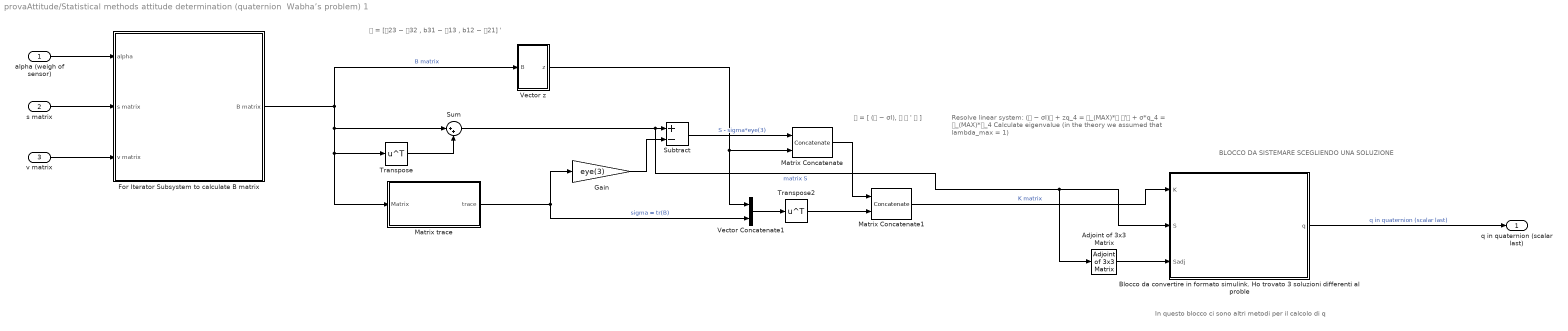
== system provaAttitude/Statistical methods attitude determination (quaternion  Wabha’s problem) 1 ==
  note: In questo blocco ci sono altri metodi per il calcolo di q
  note: BLOCCO DA SISTEMARE SCEGLIENDO UNA SOLUZIONE
  note: Resolve linear system:
      | (𝑆 − σI)𝑞 + zq_4 = 𝜆_(MAX)*𝑞
      | 𝑧'𝑞 + σ*q_4 = 𝜆_(MAX)*𝑞_4
      |
      | Calculate eigenvalue (in the theory we assumed that lambda_max = 1)
  note: 𝐾 = [ (𝑆 − σI), 𝑧
      | 𝑧 ' 𝜎 ]
  note: 𝑧 = [𝑏23 − 𝑏32 , b31 − 𝑏13 , b12 − 𝑏21] '
  alpha (weigh of sensor) : Inport
  s matrix : Inport  Port=2
  v matrix : Inport  Port=3
  Adjoint of 3x3 Matrix : aerolibutil/Adjoint of 3x3 Matrix
  Blocco da convertire in formato simulink. Ho trovato 3 soluzioni differenti al proble : MATLAB Function  TreatAsAtomicUnit=on
  For Iterator Subsystem to calculate B matrix : Subsystem  TreatAsAtomicUnit=on
  Gain : Gain  Gain=eye(3)
  Matrix Concatenate : Concatenate  Mode=Multidimensional array  ConcatenateDimension=2
  Matrix Concatenate1 : Concatenate  Mode=Multidimensional array
  Matrix trace : Subsystem
  Subtract : Sum  Inputs=+-
  Sum : Sum  Inputs=|++
  Transpose : Math  Operator=transpose
  Transpose2 : Math  Operator=transpose
  Vector Concatenate1 : Concatenate
  Vector z : Subsystem
  q in quaternion (scalar last) : Outport
  wires:
  Transpose/1 -> Sum/2
  For Iterator Subsystem to calculate B matrix/1(B matrix) -> Vector z/1(B), Matrix trace/1(Matrix), Transpose/1, Sum/1  "B matrix"
  Sum/1 -> Adjoint of 3x3 Matrix/1, Blocco da convertire in formato simulink. Ho trovato 3 soluzioni differenti al proble/2(S), Subtract/1  "matrix S"
  Gain/1 -> Subtract/2
  Matrix trace/1(trace) -> Vector Concatenate1/2, Gain/1  "sigma = tr(B)"
  Matrix Concatenate/1 -> Matrix Concatenate1/1
  Vector Concatenate1/1 -> Transpose2/1
  Vector z/1(z) -> Vector Concatenate1/1, Matrix Concatenate/2
  Transpose2/1 -> Matrix Concatenate1/2
  Subtract/1 -> Matrix Concatenate/1  "S - sigma*eye(3)"
  alpha (weigh of sensor)/1 -> For Iterator Subsystem to calculate B matrix/1(alpha)
  v matrix/1 -> For Iterator Subsystem to calculate B matrix/3(v matrix)
  s matrix/1 -> For Iterator Subsystem to calculate B matrix/2(s matrix)
  Blocco da convertire in formato simulink. Ho trovato 3 soluzioni differenti al proble/1(q) -> q in quaternion (scalar last)/1  "q in quaternion (scalar last)"
  Adjoint of 3x3 Matrix/1 -> Blocco da convertire in formato simulink. Ho trovato 3 soluzioni differenti al proble/3(Sadj)
  Matrix Concatenate1/1 -> Blocco da convertire in formato simulink. Ho trovato 3 soluzioni differenti al proble/1(K)  "K matrix"

== system provaAttitude/Sun Position in Earth Centred Equatorial Inertial RF ==
  1 day in second1 : Constant  Value=3600*24
  Clock1 : Clock
  Constant2 : Constant  Value=MJD2000_initial
  Constant3 : Constant  Value=[1 0 0; 0 cos(epsilon) -sin(epsilon); 0 sin(epsilon) cos(epsilon)]
  Divide1 : Product  Inputs=*/
  Gain1 : Gain  Gain=-1
  MATLAB Function1 : MATLAB Function  TreatAsAtomicUnit=on
  Matrix Multiply1 : Product  Multiplication=Matrix(*)
  Sum1 : Sum  Inputs=|++
  S_EarthSun_N : Outport
  wires:
  1 day in second1/1 -> Divide1/2
  Sum1/1 -> MATLAB Function1/1(MJD2000)  "mjd2000"
  Divide1/1 -> Sum1/1
  Constant3/1 -> Matrix Multiply1/1
  Matrix Multiply1/1 -> Gain1/1
  Clock1/1 -> Divide1/1
  MATLAB Function1/1(r) -> Matrix Multiply1/2
  Constant2/1 -> Sum1/2
  Gain1/1 -> S_EarthSun_N/1

== system provaAttitude/Sun sensor (Da fare) ==
  note: SUN SENSOR DA RIFINIRE, ma Utilizzabile
      | -> Modellare non rilevamento sole (esempio eclissi)
      | -> Modellare albedo terra/luna per riflessi
      | -> Sistemare distrubi basandosi su sensore reale
  DCM_B/N : Inport
  S_n : Inport  Port=2
  Band-Limited White Noise : simulink/Sources/Band-Limited White Noise  Cov=5e9*[1 1 1]  Ts=ts_sensor  seed=[23341]
  Normalize Vector1 : Subsystem
  Rotation in body frame : Product  Multiplication=Matrix(*)
  Rotation in body frame1 : Product  Multiplication=Matrix(*)
  Sum : Sum  Inputs=|++
  Zero-Order Hold : ZeroOrderHold  SampleTime=ts_sensor
  S_b unperturbed : Outport
  Perturbed data sun sensor : Outport  Port=2
  wires:
  Band-Limited White Noise/1 -> Sum/2
  DCM_B/N/1 -> Rotation in body frame/1, Rotation in body frame1/1
  S_n/1 -> Zero-Order Hold/1, Normalize Vector1/1(Vector)
  Normalize Vector1/1(Versor) -> Rotation in body frame/2
  Zero-Order Hold/1 -> Rotation in body frame1/2
  Rotation in body frame1/1 -> Sum/1
  Rotation in body frame/1 -> S_b unperturbed/1
  Sum/1 -> Perturbed data sun sensor/1

== system provaAttitude/two-body Keplerian dynamics ==
  th0 : Inport
  Constant : Constant  Value=DCM_eci_per
  Integretion of true anomaly : Subsystem
  Matrix Multiply : Product  Multiplication=Matrix(*)
  Transpose : Math  Operator=transpose
  r_perifocal : Subsystem
  r_n : Outport
  wires:
  th0/1 -> Integretion of true anomaly/1(th0)
  Integretion of true anomaly/1(th) -> r_perifocal/1(th)
  Constant/1 -> Transpose/1
  Transpose/1 -> Matrix Multiply/1
  r_perifocal/1(r_per) -> Matrix Multiply/2
  Matrix Multiply/1 -> r_n/1

== system provaAttitude/Attitude determination algebric Method with 2 sensor/Normalize Vector1 ==
  Vector : Inport
  Divide : Product  Inputs=*/
  Normalize Vector : Subsystem  AncestorBlock=LibrarySAD5/Normalize Vector1
  Versor : Outport
  wires:
  Vector/1 -> Normalize Vector/1(Vector), Divide/1
  Divide/1 -> Versor/1
  Normalize Vector/1(Norm) -> Divide/2

== system provaAttitude/Attitude determination algebric Method with 2 sensor/Normalize Vector2 ==
  Vector : Inport
  Divide : Product  Inputs=*/
  Normalize Vector : Subsystem  AncestorBlock=LibrarySAD5/Normalize Vector1
  Versor : Outport
  wires:
  Vector/1 -> Normalize Vector/1(Vector), Divide/1
  Divide/1 -> Versor/1
  Normalize Vector/1(Norm) -> Divide/2

== system provaAttitude/Attitude determination algebric Method with 2 sensor/Normalize Vector3 ==
  Vector : Inport
  Divide : Product  Inputs=*/
  Normalize Vector : Subsystem  AncestorBlock=LibrarySAD5/Normalize Vector1
  Versor : Outport
  wires:
  Vector/1 -> Normalize Vector/1(Vector), Divide/1
  Divide/1 -> Versor/1
  Normalize Vector/1(Norm) -> Divide/2

== system provaAttitude/Attitude determination algebric Method with 2 sensor/Normalize Vector4 ==
  Vector : Inport
  Divide : Product  Inputs=*/
  Normalize Vector : Subsystem  AncestorBlock=LibrarySAD5/Normalize Vector1
  Versor : Outport
  wires:
  Vector/1 -> Normalize Vector/1(Vector), Divide/1
  Divide/1 -> Versor/1
  Normalize Vector/1(Norm) -> Divide/2

== system provaAttitude/Attitude determination algebric Method with 2 sensor/Subsystem ==
  note: S1 = 𝑝;
      | 𝑠2 = (𝑝 ∧ 𝑞)/(|𝑝 ∧ 𝑞|);
      | 𝑠3 = 𝑝 ∧ 𝑠2
  versor p (body frame) : Inport
  versor q (body frame) : Inport  Port=2
  Cross Product : matrix_library/Cross Product
  Cross Product1 : matrix_library/Cross Product
  Matrix Concatenate : Concatenate  NumInputs=3  Mode=Multidimensional array  ConcatenateDimension=2
  Normalize Vector3 : Subsystem
  "Matrix S Measurements " : Outport
  wires:
  versor q (body frame)/1 -> Cross Product/2
  Normalize Vector3/1(Versor) -> Matrix Concatenate/2, Cross Product1/2  "s2"
  versor p (body frame)/1 -> Cross Product1/1, Matrix Concatenate/1, Cross Product/1  "s1"
  Cross Product/1 -> Normalize Vector3/1(Vector)
  Cross Product1/1 -> Matrix Concatenate/3  "s3"
  Matrix Concatenate/1 -> "Matrix S Measurements "/1  "Matrix of measure in body frame"

== system provaAttitude/Attitude determination algebric Method with 2 sensor/Subsystem1 ==
  versor a (body frame) : Inport
  versor b (body frame) : Inport  Port=2
  Cross Product : matrix_library/Cross Product
  Cross Product1 : matrix_library/Cross Product
  Matrix Concatenate : Concatenate  NumInputs=3  Mode=Multidimensional array  ConcatenateDimension=2
  Normalize Vector3 : Subsystem
  "Matrix V certain model " : Outport
  wires:
  versor b (body frame)/1 -> Cross Product/2
  Normalize Vector3/1(Versor) -> Matrix Concatenate/2, Cross Product1/2  "s2"
  versor a (body frame)/1 -> Cross Product1/1, Matrix Concatenate/1, Cross Product/1  "s1"
  Cross Product/1 -> Normalize Vector3/1(Vector)
  Cross Product1/1 -> Matrix Concatenate/3  "s3"
  Matrix Concatenate/1 -> "Matrix V certain model "/1  "Matrix of measure in body frame"

== system provaAttitude/Attitude determination algebric Method with 2 sensor1/Normalize Vector1 ==
  Vector : Inport
  Divide : Product  Inputs=*/
  Normalize Vector : Subsystem  AncestorBlock=LibrarySAD5/Normalize Vector1
  Versor : Outport
  wires:
  Vector/1 -> Normalize Vector/1(Vector), Divide/1
  Divide/1 -> Versor/1
  Normalize Vector/1(Norm) -> Divide/2

== system provaAttitude/Attitude determination algebric Method with 2 sensor1/Normalize Vector2 ==
  Vector : Inport
  Divide : Product  Inputs=*/
  Normalize Vector : Subsystem  AncestorBlock=LibrarySAD5/Normalize Vector1
  Versor : Outport
  wires:
  Vector/1 -> Normalize Vector/1(Vector), Divide/1
  Divide/1 -> Versor/1
  Normalize Vector/1(Norm) -> Divide/2

== system provaAttitude/Attitude determination algebric Method with 2 sensor1/Normalize Vector3 ==
  Vector : Inport
  Divide : Product  Inputs=*/
  Normalize Vector : Subsystem  AncestorBlock=LibrarySAD5/Normalize Vector1
  Versor : Outport
  wires:
  Vector/1 -> Normalize Vector/1(Vector), Divide/1
  Divide/1 -> Versor/1
  Normalize Vector/1(Norm) -> Divide/2

== system provaAttitude/Attitude determination algebric Method with 2 sensor1/Normalize Vector4 ==
  Vector : Inport
  Divide : Product  Inputs=*/
  Normalize Vector : Subsystem  AncestorBlock=LibrarySAD5/Normalize Vector1
  Versor : Outport
  wires:
  Vector/1 -> Normalize Vector/1(Vector), Divide/1
  Divide/1 -> Versor/1
  Normalize Vector/1(Norm) -> Divide/2

== system provaAttitude/Attitude determination algebric Method with 2 sensor1/Subsystem ==
  note: S1 = 𝑝;
      | 𝑠2 = (𝑝 ∧ 𝑞)/(|𝑝 ∧ 𝑞|);
      | 𝑠3 = 𝑝 ∧ 𝑠2
  versor p (body frame) : Inport
  versor q (body frame) : Inport  Port=2
  Cross Product : matrix_library/Cross Product
  Cross Product1 : matrix_library/Cross Product
  Matrix Concatenate : Concatenate  NumInputs=3  Mode=Multidimensional array  ConcatenateDimension=2
  Normalize Vector3 : Subsystem
  "Matrix S Measurements " : Outport
  wires:
  versor q (body frame)/1 -> Cross Product/2
  Normalize Vector3/1(Versor) -> Matrix Concatenate/2, Cross Product1/2  "s2"
  versor p (body frame)/1 -> Cross Product1/1, Matrix Concatenate/1, Cross Product/1  "s1"
  Cross Product/1 -> Normalize Vector3/1(Vector)
  Cross Product1/1 -> Matrix Concatenate/3  "s3"
  Matrix Concatenate/1 -> "Matrix S Measurements "/1  "Matrix of measure in body frame"

== system provaAttitude/Attitude determination algebric Method with 2 sensor1/Subsystem1 ==
  versor a (body frame) : Inport
  versor b (body frame) : Inport  Port=2
  Cross Product : matrix_library/Cross Product
  Cross Product1 : matrix_library/Cross Product
  Matrix Concatenate : Concatenate  NumInputs=3  Mode=Multidimensional array  ConcatenateDimension=2
  Normalize Vector3 : Subsystem
  "Matrix V certain model " : Outport
  wires:
  versor b (body frame)/1 -> Cross Product/2
  Normalize Vector3/1(Versor) -> Matrix Concatenate/2, Cross Product1/2  "s2"
  versor a (body frame)/1 -> Cross Product1/1, Matrix Concatenate/1, Cross Product/1  "s1"
  Cross Product/1 -> Normalize Vector3/1(Vector)
  Cross Product1/1 -> Matrix Concatenate/3  "s3"
  Matrix Concatenate/1 -> "Matrix V certain model "/1  "Matrix of measure in body frame"

== system provaAttitude/Calculation of disturbance torque/M of Solar Pressure ==
  DCM_B/N : Inport
  EarthSat_n vector : Inport  Port=2
  SunEarth_n vector : Inport  Port=3
  Calculation of F_i : Subsystem
  Constant : Constant  Value=BODY
  Matrix Multiply : Product  Multiplication=Matrix(*)
  Normalize Vector : Subsystem
  Subtract : Sum  Inputs=--
  Torque calculation : Subsystem
  M_SRP : Outport
  wires:
  Calculation of F_i/1(F_i matrix) -> Torque calculation/1(F_i Matrix)
  EarthSat_n vector/1 -> Subtract/1
  Constant/1 -> Calculation of F_i/1(body versor matrix)
  Normalize Vector/1(Versor) -> Calculation of F_i/2(Sb_vector1)
  Torque calculation/1(M_SRP) -> M_SRP/1
  SunEarth_n vector/1 -> Subtract/2
  Subtract/1 -> Matrix Multiply/2  "SatSun_vector inertial"
  Matrix Multiply/1 -> Normalize Vector/1(Vector)
  DCM_B/N/1 -> Matrix Multiply/1

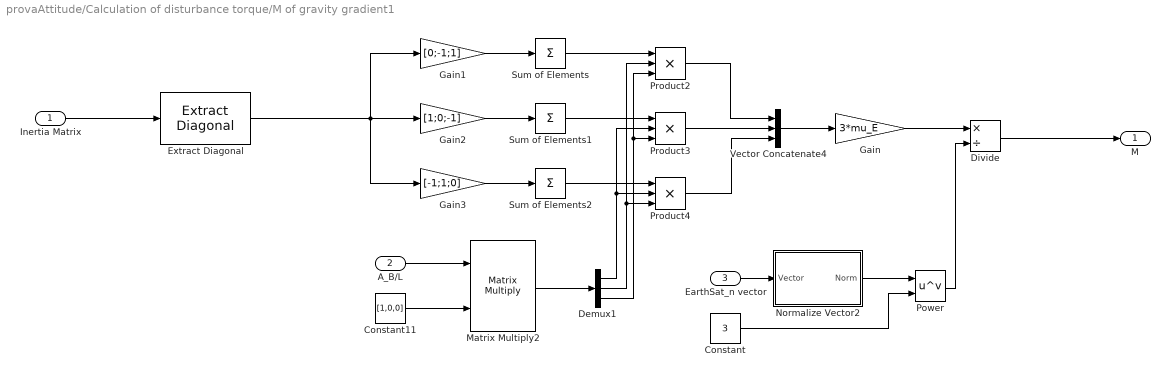
== system provaAttitude/Calculation of disturbance torque/M of gravity gradient1 ==
  Inertia Matrix : Inport
  A_B/L : Inport  Port=2
  EarthSat_n vector : Inport  Port=3
  Constant : Constant  Value=3
  Constant11 : Constant  Value=[1,0,0]
  Demux1 : Demux  Outputs=3
  Divide : Product  Inputs=*/
  Extract Diagonal : matrix_library/Extract Diagonal
      settings: LibrarySourceBlock=|
      | simulink/Matrix
      | Operations/Extract Diagonal
  Gain : Gain  Gain=3*mu_E
  Gain1 : Gain  Gain=[0;-1;1]
  Gain2 : Gain  Gain=[1;0;-1]
  Gain3 : Gain  Gain=[-1;1;0]
  Matrix Multiply2 : Product  Multiplication=Matrix(*)
  Normalize Vector2 : Subsystem  AncestorBlock=LibrarySAD5/Normalize Vector1
  Power : Math  Operator=pow
  Product2 : Product  Inputs=3
  Product3 : Product  Inputs=3
  Product4 : Product  Inputs=3
  Sum of Elements : Sum  Inputs=+
  Sum of Elements1 : Sum  Inputs=+
  Sum of Elements2 : Sum  Inputs=+
  Vector Concatenate4 : Concatenate  NumInputs=3
  M : Outport
  wires:
  Demux1/3 -> Product2/3, Product3/3
  Product2/1 -> Vector Concatenate4/1
  Matrix Multiply2/1 -> Demux1/1
  Product4/1 -> Vector Concatenate4/3
  Product3/1 -> Vector Concatenate4/2
  Demux1/1 -> Product4/2, Product3/2
  Constant11/1 -> Matrix Multiply2/2
  Demux1/2 -> Product4/3, Product2/2
  A_B/L/1 -> Matrix Multiply2/1
  Vector Concatenate4/1 -> Gain/1
  Gain1/1 -> Sum of Elements/1
  Gain2/1 -> Sum of Elements1/1
  Gain3/1 -> Sum of Elements2/1
  Sum of Elements/1 -> Product2/1
  Sum of Elements1/1 -> Product3/1
  Sum of Elements2/1 -> Product4/1
  Inertia Matrix/1 -> Extract Diagonal/1
  Gain/1 -> Divide/1
  EarthSat_n vector/1 -> Normalize Vector2/1(Vector)
  Power/1 -> Divide/2
  Constant/1 -> Power/2
  Normalize Vector2/1(Norm) -> Power/1
  Divide/1 -> M/1
  Extract Diagonal/1 -> Gain1/1, Gain2/1, Gain3/1

== system provaAttitude/Calculation of disturbance torque/Magnetic Torque ==
  j_b : Inport
  B_b : Inport  Port=2
  Cross Product : matrix_library/Cross Product
  M_b : Outport
  wires:
  Cross Product/1 -> M_b/1
  j_b/1 -> Cross Product/1
  B_b/1 -> Cross Product/2

== system provaAttitude/Create matrix to statistical method/Normalize Vector1 ==
  Vector : Inport
  Divide : Product  Inputs=*/
  Normalize Vector : Subsystem  AncestorBlock=LibrarySAD5/Normalize Vector1
  Versor : Outport
  wires:
  Vector/1 -> Normalize Vector/1(Vector), Divide/1
  Divide/1 -> Versor/1
  Normalize Vector/1(Norm) -> Divide/2

== system provaAttitude/Create matrix to statistical method/Normalize Vector2 ==
  Vector : Inport
  Divide : Product  Inputs=*/
  Normalize Vector : Subsystem  AncestorBlock=LibrarySAD5/Normalize Vector1
  Versor : Outport
  wires:
  Vector/1 -> Normalize Vector/1(Vector), Divide/1
  Divide/1 -> Versor/1
  Normalize Vector/1(Norm) -> Divide/2

== system provaAttitude/Create matrix to statistical method/Normalize Vector3 ==
  Vector : Inport
  Divide : Product  Inputs=*/
  Normalize Vector : Subsystem  AncestorBlock=LibrarySAD5/Normalize Vector1
  Versor : Outport
  wires:
  Vector/1 -> Normalize Vector/1(Vector), Divide/1
  Divide/1 -> Versor/1
  Normalize Vector/1(Norm) -> Divide/2

== system provaAttitude/Create matrix to statistical method/Normalize Vector4 ==
  Vector : Inport
  Divide : Product  Inputs=*/
  Normalize Vector : Subsystem  AncestorBlock=LibrarySAD5/Normalize Vector1
  Versor : Outport
  wires:
  Vector/1 -> Normalize Vector/1(Vector), Divide/1
  Divide/1 -> Versor/1
  Normalize Vector/1(Norm) -> Divide/2

== system provaAttitude/Create matrix to statistical method1/Normalize Vector1 ==
  Vector : Inport
  Divide : Product  Inputs=*/
  Normalize Vector : Subsystem  AncestorBlock=LibrarySAD5/Normalize Vector1
  Versor : Outport
  wires:
  Vector/1 -> Normalize Vector/1(Vector), Divide/1
  Divide/1 -> Versor/1
  Normalize Vector/1(Norm) -> Divide/2

== system provaAttitude/Create matrix to statistical method1/Normalize Vector2 ==
  Vector : Inport
  Divide : Product  Inputs=*/
  Normalize Vector : Subsystem  AncestorBlock=LibrarySAD5/Normalize Vector1
  Versor : Outport
  wires:
  Vector/1 -> Normalize Vector/1(Vector), Divide/1
  Divide/1 -> Versor/1
  Normalize Vector/1(Norm) -> Divide/2

== system provaAttitude/Create matrix to statistical method1/Normalize Vector3 ==
  Vector : Inport
  Divide : Product  Inputs=*/
  Normalize Vector : Subsystem  AncestorBlock=LibrarySAD5/Normalize Vector1
  Versor : Outport
  wires:
  Vector/1 -> Normalize Vector/1(Vector), Divide/1
  Divide/1 -> Versor/1
  Normalize Vector/1(Norm) -> Divide/2
